simulink model "DroopandPImodel"  (R2024b)
settings: Solver=VariableStepAuto  StartTime=0.0  StopTime=10  RelTol=1e-3
values from neighbouring files (symbols this model uses):
  c = 160e-6    (= 0.00016)    [ParamTestSimulationDroop.m]    (also in ParamTestSimulatitestFirstandPI.m)
  deltaV = vrated*0.05    (= 5.5)    [ParamTestSimulationDroop.m]
  deltaW = 0.05*wrated    (= 18.8495559215)    [ParamTestSimulationDroop.m]
  Kp_currentLoop = X*r    (= 0.5)    [ParamTestSimulationDroop.m]    (also in ParamTestSimulatitestFirstandPI.m)
  Kp_voltageLoop = Xvoltage/Rc    (= 0.005)    [ParamTestSimulationDroop.m]    (also in ParamTestSimulatitestFirstandPI.m)
  l = 300e-6    (= 0.0003)    [ParamTestSimulationDroop.m]    (also in ParamTestSimulatitestFirstandPI.m)
  m = deltaW/Pnominal    (= 0.00628318530718)    [ParamTestSimulationDroop.m]
  n = deltaV/Qnominal    (= 0.011)    [ParamTestSimulationDroop.m]
  Pnominal = 3000    [ParamTestSimulationDroop.m]
  Qnominal = 500    [ParamTestSimulationDroop.m]
  r = 0.1    [ParamTestSimulationDroop.m]    (also in ParamTestSimulatitestFirstandPI.m)
  Rc = 1e3    (= 1000)    [ParamTestSimulationDroop.m]    (also in ParamTestSimulatitestFirstandPI.m)
  T32 = sqrt(2/3)*[1 0;-1/2 sqrt(3)/2;-1/2 -sqrt(3)/2]    [ParamTestSimulationDroop.m]    (also in ParamTestSimulatitestFirstandPI.m)
  towI_currentLoop = tow_currnet    (= 0.003)    [ParamTestSimulationDroop.m]    (also in ParamTestSimulatitestFirstandPI.m)
  towI_voltageLoop = tow_voltage    (= 0.16)    [ParamTestSimulationDroop.m]    (also in ParamTestSimulatitestFirstandPI.m)
  vrated = 110    [ParamTestSimulationDroop.m]
  wrated = 2*pi*60    (= 376.991118431)    [ParamTestSimulationDroop.m]
undefined symbols (not defined in the file or in its folder): DiscIntNeverNeededParam
libraries: spsThreePhaseSeriesRLCBranchLib x6, spsControlledVoltageSourceLib x3, spsThreePhaseVIMeasurementLib x2, spsGroundLib x1, sps_lib x1
settings Model: Creator=manip  LastModifiedBy=rashi
settings SolverCC: AlgebraicLoopSolver=TrustRegion
settings DebuggingCC: UnconnectedInputMsg=warning  UnconnectedOutputMsg=warning  UnconnectedLineMsg=warning
settings ModelReferenceCC: EnableRefExpFcnMdlSchedulingChecks=on
settings RTWCC: GPUComputeCapability=3.5

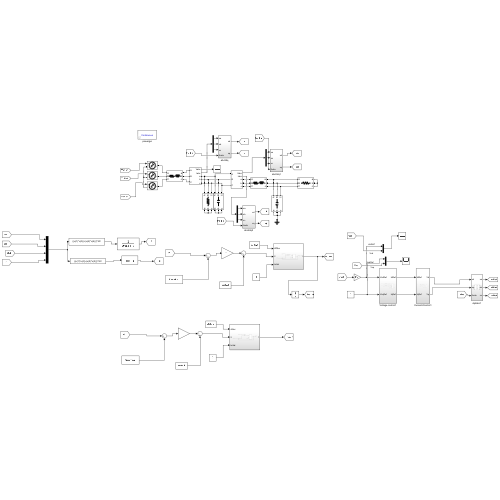
[thumbnail: Simulink's stored preview of the top-level diagram]
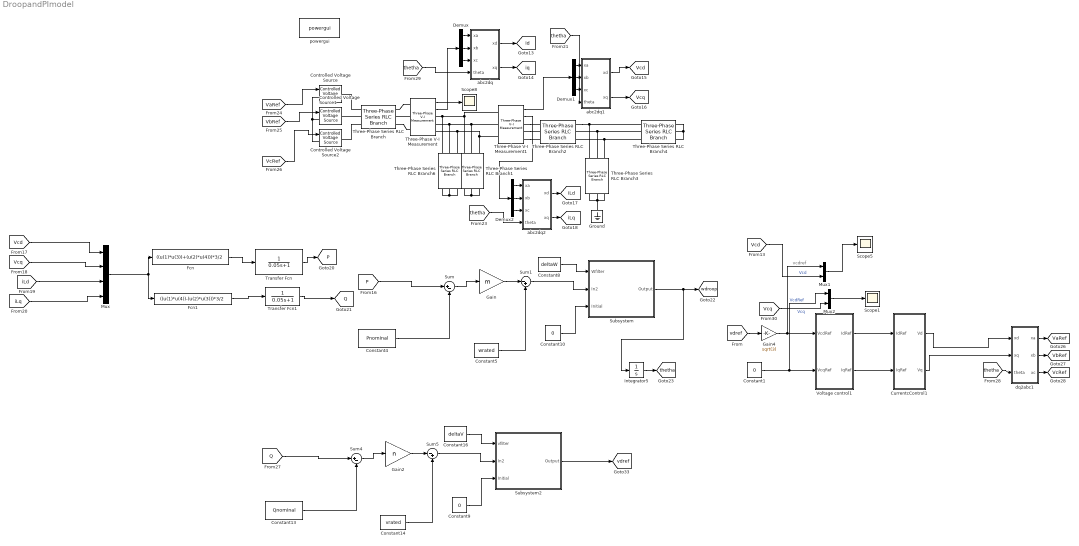
== system DroopandPImodel ==
  note: vcdref
  Constant1 : Constant  Value=0
  Constant10 : Constant  Value=0
  Constant13 : Constant  Value=Qnominal
  Constant14 : Constant  Value=vrated
  Constant16 : Constant  Value=deltaV
  Constant4 : Constant  Value=Pnominal
  Constant5 : Constant  Value=wrated
  Constant8 : Constant  Value=deltaW
  Constant9 : Constant  Value=0
  Controlled Voltage Source : spsControlledVoltageSourceLib/Controlled Voltage Source  Initialize=on  Source_Type=AC  Amplitude=0  Phase=0  Frequency=0  Measurements=None
  Controlled Voltage Source1 : spsControlledVoltageSourceLib/Controlled Voltage Source  Initialize=on  Source_Type=AC  Amplitude=0  Phase=0  Frequency=0  Measurements=None
  Controlled Voltage Source2 : spsControlledVoltageSourceLib/Controlled Voltage Source  Initialize=on  Source_Type=AC  Amplitude=0  Phase=0  Frequency=0  Measurements=None
  CurrentcControl1 : Subsystem
  Demux : Demux  Outputs=3
  Demux1 : Demux  Outputs=3
  Demux2 : Demux  Outputs=3
  Fcn : Fcn  Expr=((u(1)*u(3))+(u(2)*u(4)))*3/2
  Fcn1 : Fcn  Expr=((u(1)*u(4))-(u(2)*u(3)))*3/2
  Gain : Gain  Gain=m
  Gain2 : Gain  Gain=n
  Gain4 : Gain  Gain=sqrt(3)
  Ground : spsGroundLib/Ground  LConnTagsString=a
  Integrator5 : Integrator
  Mux : Mux
  Mux1 : Mux  Inputs=2
  Mux2 : Mux  Inputs=2
  Scope1 : Scope
  Scope5 : Scope
  Scope8 : Scope
  Subsystem : Subsystem
  Subsystem2 : Subsystem
  Sum : Sum  Inputs=|+-
  Sum1 : Sum  Inputs=|-+
  Sum4 : Sum  Inputs=|+-
  Sum5 : Sum  Inputs=|-+
  Three-Phase Series RLC Branch : spsThreePhaseSeriesRLCBranchLib/Three-Phase Series RLC Branch  LConnTagsString=A|B|C  RConnTagsString=A|B|C  BranchType=RL  Resistance=r  Inductance=l  Capacitance=1e-6  Measurements=None
  Three-Phase Series RLC Branch1 : spsThreePhaseSeriesRLCBranchLib/Three-Phase Series RLC Branch  LConnTagsString=A|B|C  RConnTagsString=A|B|C  BranchType=C  Resistance=r  Inductance=l  Capacitance=c  Measurements=None
  Three-Phase Series RLC Branch2 : spsThreePhaseSeriesRLCBranchLib/Three-Phase Series RLC Branch  LConnTagsString=A|B|C  RConnTagsString=A|B|C  BranchType=RL  Resistance=1  Inductance=4e-3  Capacitance=1e-6  Measurements=None
  Three-Phase Series RLC Branch3 : spsThreePhaseSeriesRLCBranchLib/Three-Phase Series RLC Branch  LConnTagsString=A|B|C  RConnTagsString=A|B|C  BranchType=C  Resistance=r  Inductance=l  Capacitance=1e-6  Measurements=None
  Three-Phase Series RLC Branch4 : spsThreePhaseSeriesRLCBranchLib/Three-Phase Series RLC Branch  LConnTagsString=A|B|C  RConnTagsString=A|B|C  BranchType=R  Resistance=50  Inductance=4e-3  Capacitance=1e-6  Measurements=None
  Three-Phase Series RLC Branch6 : spsThreePhaseSeriesRLCBranchLib/Three-Phase Series RLC Branch  LConnTagsString=A|B|C  RConnTagsString=A|B|C  BranchType=R  Resistance=Rc  Inductance=l  Capacitance=c  Measurements=None
  Three-Phase V-I Measurement : spsThreePhaseVIMeasurementLib/Three-Phase V-I Measurement  VoltageMeasurement=phase-to-ground  SetLabelV=off  LabelV=Vabc  Vpu=off  VpuLL=off  CurrentMeasurement=yes  SetLabelI=off  LabelI=Iabc  Ipu=off  Pbase=100e6  Vbase=500e3  OutputType=Complex  PhasorSimulation=off  PSBequivalent=0
  Three-Phase V-I Measurement1 : spsThreePhaseVIMeasurementLib/Three-Phase V-I Measurement  VoltageMeasurement=phase-to-ground  SetLabelV=off  LabelV=Vabc  Vpu=off  VpuLL=off  CurrentMeasurement=yes  SetLabelI=off  LabelI=Iabc  Ipu=off  Pbase=100e6  Vbase=500e3  OutputType=Complex  PhasorSimulation=off  PSBequivalent=0
  Transfer Fcn : TransferFcn  Denominator=[0.05 1]
  Transfer Fcn1 : TransferFcn  Denominator=[0.05 1]
  Voltage control1 : Subsystem
  abc2dq : Subsystem
  abc2dq1 : Subsystem
  abc2dq2 : Subsystem
  dq2abc1 : Subsystem
  powergui : sps_lib/powergui  Priority=1  SimulationMode=Continuous  SampleTime=50e-6  frequency=60  Iterations=50  frequencyindice=0  Pbase=100e6  ErrMax=1e-4  UnitsV=kV  UnitsW=MW  buscounter=0  FunctionMessages=off  echomessages=off  EnableUseOfTLC=off  CurrentSourceSwitches=off  DisableSnubberDevices=off  DisableRonSwitches=off  DisableVfSwitches=off  DisplayEquations=off  AutomaticDiscreteSolvers=off  SolverType=Tustin/Backward Euler (TBE)  Interpol=off  ExternalGateDelay=off  methode=off  Ts=100  x0status=blocks  SPID=on  SwTol=0  HookPort=off  NonlinearTolerance=1e-4  nMaxIteration=100  ContinueOnMaxIteration=off  RestoreLinks=warning  ResistiveCurrentMeasurement=off  Frange=[0:2:500]  Ylog=off  Xlog=on  ShowGrid=off  save=off  variable=ZData  structure=0  ZoomFFT=off  StartTime=0.0  cycles=1  DisplayStyle=1  fundamental=60  FreqAxis=off  MaxFrequency=1000  frequencyindicesteady=1  RmsSteady=1  display=off
  tag scope: P=global, Q=global, VaRef=global, VbRef=global, VcRef=global, Vcd=global, Vcq=global, iLd=global, iLq=global, id=global, iq=global, thetha=global, vdref=global, wdroop=global
  wires:
  Demux/1 -> abc2dq/1(xa)
  Demux/2 -> abc2dq/2(xb)
  Demux/3 -> abc2dq/3(xc)
  Three-Phase V-I Measurement/2 -> Demux/1
  abc2dq/1(xd) -> [id]
  abc2dq/2(xq) -> [iq]
  Three-Phase V-I Measurement1/1 -> Demux1/1
  Demux1/3 -> abc2dq1/3(xc)
  Demux1/2 -> abc2dq1/2(xb)
  Demux1/1 -> abc2dq1/1(xa)
  abc2dq1/1(xd) -> [Vcd]
  abc2dq1/2(xq) -> [Vcq]
  abc2dq2/2(xq) -> [iLq]
  abc2dq2/1(xd) -> [iLd]
  Three-Phase V-I Measurement1/2 -> Demux2/1
  Demux2/2 -> abc2dq2/2(xb)
  Demux2/3 -> abc2dq2/3(xc)
  Demux2/1 -> abc2dq2/1(xa)
  [iLd] -> Mux/3
  [iLq] -> Mux/4
  Mux/1 -> Fcn/1, Fcn1/1
  Constant4/1 -> Sum/2
  Sum/1 -> Gain/1
  Gain/1 -> Sum1/1
  Constant5/1 -> Sum1/2
  Sum1/1 -> Subsystem/2(In2)
  [VaRef] -> Controlled Voltage Source/1
  [VcRef] -> Controlled Voltage Source2/1
  dq2abc1/3(xc) -> [VcRef]
  CurrentcControl1/1(Vd) -> dq2abc1/1(xd)
  dq2abc1/2(xb) -> [VbRef]
  Constant1/1 -> Mux2/1, Voltage control1/2(VcqRef)
  dq2abc1/1(xa) -> [VaRef]
  CurrentcControl1/2(Vq) -> dq2abc1/2(xq)
  Subsystem/1(Output) -> Integrator5/1, [wdroop]
  Constant8/1 -> Subsystem/1(Wfilter)
  [VbRef] -> Controlled Voltage Source1/1
  [Vcd] -> Mux/1
  [Vcq] -> Mux/2
  Transfer Fcn/1 -> [P]
  Fcn/1 -> Transfer Fcn/1
  Fcn1/1 -> Transfer Fcn1/1
  Transfer Fcn1/1 -> [Q]
  [thetha] -> dq2abc1/3(theta)
  [thetha] -> abc2dq2/4(theta)
  Constant10/1 -> Subsystem/3(Initial)
  [P] -> Sum/1
  Constant9/1 -> Subsystem2/3(Initial)
  Constant16/1 -> Subsystem2/1(vfilter)
  Constant14/1 -> Sum5/2
  Constant13/1 -> Sum4/2
  Gain2/1 -> Sum5/1
  Sum5/1 -> Subsystem2/2(In2)
  Subsystem2/1(Output) -> [vdref]
  Sum4/1 -> Gain2/1
  [Q] -> Sum4/1
  Gain4/1 -> Voltage control1/1(VcdRef), Mux1/1  "VcdRef"
  [thetha] -> abc2dq/4(theta)
  [thetha] -> abc2dq1/4(theta)
  [vdref] -> Gain4/1
  Voltage control1/2(IqRef) -> CurrentcControl1/2(IqRef)
  Voltage control1/1(IdRef) -> CurrentcControl1/1(IdRef)
  [Vcd] -> Mux1/2  "Vcd"
  Mux2/1 -> Scope1/1
  [Vcq] -> Mux2/2  "Vcq"
  Mux1/1 -> Scope5/1
  Three-Phase V-I Measurement/1 -> Scope8/1
  Integrator5/1 -> [thetha]
  connections:
  Controlled Voltage Source1/LConn1 -- Controlled Voltage Source/LConn1 -- Controlled Voltage Source2/LConn1
  Three-Phase Series RLC Branch/LConn1 -- Controlled Voltage Source/RConn1
  Three-Phase Series RLC Branch/LConn2 -- Controlled Voltage Source1/RConn1
  Three-Phase Series RLC Branch/LConn3 -- Controlled Voltage Source2/RConn1
  Three-Phase V-I Measurement/LConn1 -- Three-Phase Series RLC Branch/RConn1
  Three-Phase V-I Measurement/LConn2 -- Three-Phase Series RLC Branch/RConn2
  Three-Phase Series RLC Branch/RConn3 -- Three-Phase V-I Measurement/LConn3
  Three-Phase Series RLC Branch1/RConn3 -- Three-Phase Series RLC Branch1/RConn2 -- Three-Phase Series RLC Branch1/RConn1
  Three-Phase Series RLC Branch1/LConn1 -- Three-Phase V-I Measurement1/LConn1 -- Three-Phase Series RLC Branch6/LConn1 -- Three-Phase V-I Measurement/RConn1
  Three-Phase V-I Measurement/RConn2 -- Three-Phase Series RLC Branch6/LConn2 -- Three-Phase V-I Measurement1/LConn2 -- Three-Phase Series RLC Branch1/LConn2
  Three-Phase V-I Measurement/RConn3 -- Three-Phase Series RLC Branch6/LConn3 -- Three-Phase V-I Measurement1/LConn3 -- Three-Phase Series RLC Branch1/LConn3
  Three-Phase V-I Measurement1/RConn1 -- Three-Phase Series RLC Branch2/LConn1
  Three-Phase V-I Measurement1/RConn2 -- Three-Phase Series RLC Branch2/LConn2
  Three-Phase V-I Measurement1/RConn3 -- Three-Phase Series RLC Branch2/LConn3
  Three-Phase Series RLC Branch3/RConn2 -- Three-Phase Series RLC Branch3/RConn3 -- Ground/LConn1 -- Three-Phase Series RLC Branch3/RConn1
  Three-Phase Series RLC Branch2/RConn1 -- Three-Phase Series RLC Branch3/LConn1 -- Three-Phase Series RLC Branch4/LConn1
  Three-Phase Series RLC Branch3/LConn2 -- Three-Phase Series RLC Branch2/RConn2 -- Three-Phase Series RLC Branch4/LConn2
  Three-Phase Series RLC Branch3/LConn3 -- Three-Phase Series RLC Branch4/LConn3 -- Three-Phase Series RLC Branch2/RConn3
  Three-Phase Series RLC Branch6/RConn3 -- Three-Phase Series RLC Branch6/RConn2 -- Three-Phase Series RLC Branch6/RConn1
  Three-Phase Series RLC Branch4/RConn1 -- Three-Phase Series RLC Branch4/RConn2 -- Three-Phase Series RLC Branch4/RConn3

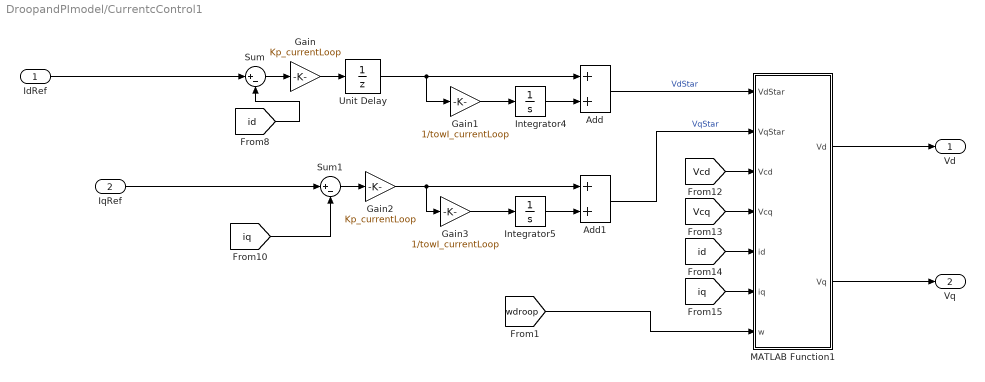
== system DroopandPImodel/CurrentcControl1 ==
  IdRef : Inport
  IqRef : Inport  Port=2
  Add : Sum
  Add1 : Sum
  Gain : Gain  Gain=Kp_currentLoop
  Gain1 : Gain  Gain=1/towI_currentLoop
  Gain2 : Gain  Gain=Kp_currentLoop
  Gain3 : Gain  Gain=1/towI_currentLoop
  Integrator4 : Integrator
  Integrator5 : Integrator
  MATLAB Function1 : MATLAB Function  TreatAsAtomicUnit=on
  Sum : Sum  Inputs=|+-
  Sum1 : Sum  Inputs=|+-
  Unit Delay : UnitDelay  SampleTime=1e-6  HasFrameUpgradeWarning=on
  Vd : Outport
  Vq : Outport  Port=2
  wires:
  [wdroop] -> MATLAB Function1/7(w)
  [iq] -> Sum1/2
  Add/1 -> MATLAB Function1/1(VdStar)  "VdStar"
  [Vcq] -> MATLAB Function1/4(Vcq)
  Gain2/1 -> Gain3/1, Add1/1
  IdRef/1 -> Sum/1
  [id] -> MATLAB Function1/5(id)
  Sum1/1 -> Gain2/1
  Gain3/1 -> Integrator5/1
  Sum/1 -> Gain/1
  IqRef/1 -> Sum1/1
  Add1/1 -> MATLAB Function1/2(VqStar)  "VqStar"
  Integrator5/1 -> Add1/2
  MATLAB Function1/2(Vq) -> Vq/1
  Gain/1 -> Unit Delay/1
  Integrator4/1 -> Add/2
  [Vcd] -> MATLAB Function1/3(Vcd)
  Gain1/1 -> Integrator4/1
  [id] -> Sum/2
  [iq] -> MATLAB Function1/6(iq)
  MATLAB Function1/1(Vd) -> Vd/1
  Unit Delay/1 -> Gain1/1, Add/1

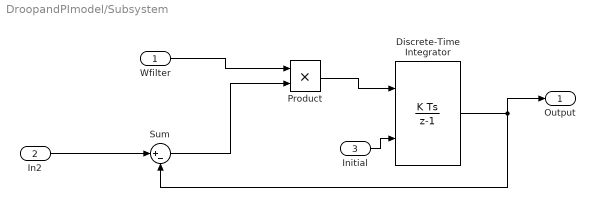
== system DroopandPImodel/Subsystem ==
  Wfilter : Inport
  In2 : Inport  Port=2
  Initial : Inport  Port=3
  Discrete-Time Integrator : DiscreteIntegrator  InitialConditionSource=external  SampleTime=1e-5  ICPrevOutput=DiscIntNeverNeededParam  ICPrevScaledInput=DiscIntNeverNeededParam
  Product : Product
  Sum : Sum  Inputs=|+-
  Output : Outport
  wires:
  Wfilter/1 -> Product/1
  In2/1 -> Sum/1
  Sum/1 -> Product/2
  Product/1 -> Discrete-Time Integrator/1
  Discrete-Time Integrator/1 -> Output/1, Sum/2
  Initial/1 -> Discrete-Time Integrator/2

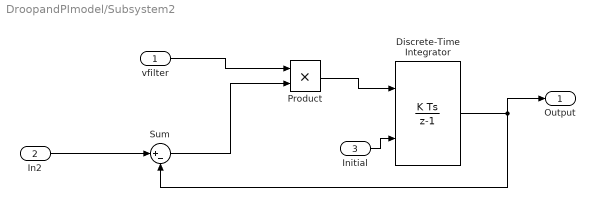
== system DroopandPImodel/Subsystem2 ==
  vfilter : Inport
  In2 : Inport  Port=2
  Initial : Inport  Port=3
  Discrete-Time Integrator : DiscreteIntegrator  InitialConditionSource=external  SampleTime=1e-5  ICPrevOutput=DiscIntNeverNeededParam  ICPrevScaledInput=DiscIntNeverNeededParam
  Product : Product
  Sum : Sum  Inputs=|+-
  Output : Outport
  wires:
  vfilter/1 -> Product/1
  In2/1 -> Sum/1
  Sum/1 -> Product/2
  Product/1 -> Discrete-Time Integrator/1
  Discrete-Time Integrator/1 -> Output/1, Sum/2
  Initial/1 -> Discrete-Time Integrator/2

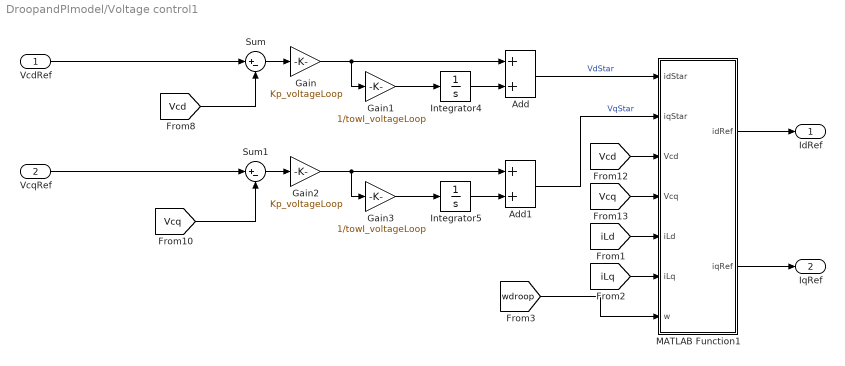
== system DroopandPImodel/Voltage control1 ==
  VcdRef : Inport
  VcqRef : Inport  Port=2
  Add : Sum
  Add1 : Sum
  Gain : Gain  Gain=Kp_voltageLoop
  Gain1 : Gain  Gain=1/towI_voltageLoop
  Gain2 : Gain  Gain=Kp_voltageLoop
  Gain3 : Gain  Gain=1/towI_voltageLoop
  Integrator4 : Integrator
  Integrator5 : Integrator
  MATLAB Function1 : MATLAB Function  TreatAsAtomicUnit=on
  Sum : Sum  Inputs=|+-
  Sum1 : Sum  Inputs=|+-
  IdRef : Outport
  IqRef : Outport  Port=2
  wires:
  Gain/1 -> Gain1/1, Add/1
  Integrator5/1 -> Add1/2
  VcqRef/1 -> Sum1/1
  Sum/1 -> Gain/1
  Gain3/1 -> Integrator5/1
  [iLd] -> MATLAB Function1/5(iLd)
  Sum1/1 -> Gain2/1
  VcdRef/1 -> Sum/1
  [Vcq] -> MATLAB Function1/4(Vcq)
  Gain2/1 -> Gain3/1, Add1/1
  [Vcd] -> Sum/2
  [iLq] -> MATLAB Function1/6(iLq)
  [wdroop] -> MATLAB Function1/7(w)
  Gain1/1 -> Integrator4/1
  [Vcq] -> Sum1/2
  Add1/1 -> MATLAB Function1/2(iqStar)  "VqStar"
  [Vcd] -> MATLAB Function1/3(Vcd)
  Add/1 -> MATLAB Function1/1(idStar)  "VdStar"
  Integrator4/1 -> Add/2
  MATLAB Function1/1(idRef) -> IdRef/1
  MATLAB Function1/2(iqRef) -> IqRef/1

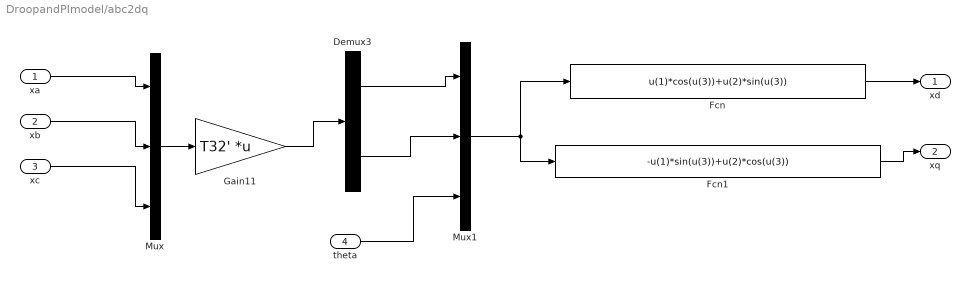
== system DroopandPImodel/abc2dq ==
  xa : Inport
  xb : Inport  Port=2
  xc : Inport  Port=3
  theta : Inport  Port=4
  Demux3 : Demux  Outputs=2
  Fcn : Fcn  Expr=u(1)*cos(u(3))+u(2)*sin(u(3))
  Fcn1 : Fcn  Expr=-u(1)*sin(u(3))+u(2)*cos(u(3))
  Gain11 : Gain  Gain=T32'  Multiplication=Matrix(K*u)
  Mux : Mux  Inputs=3
  Mux1 : Mux  Inputs=3
  xd : Outport
  xq : Outport  Port=2
  wires:
  Fcn1/1 -> xq/1
  theta/1 -> Mux1/3
  xb/1 -> Mux/2
  Mux/1 -> Gain11/1
  Gain11/1 -> Demux3/1
  xc/1 -> Mux/3
  Mux1/1 -> Fcn/1, Fcn1/1
  Fcn/1 -> xd/1
  xa/1 -> Mux/1
  Demux3/1 -> Mux1/1
  Demux3/2 -> Mux1/2

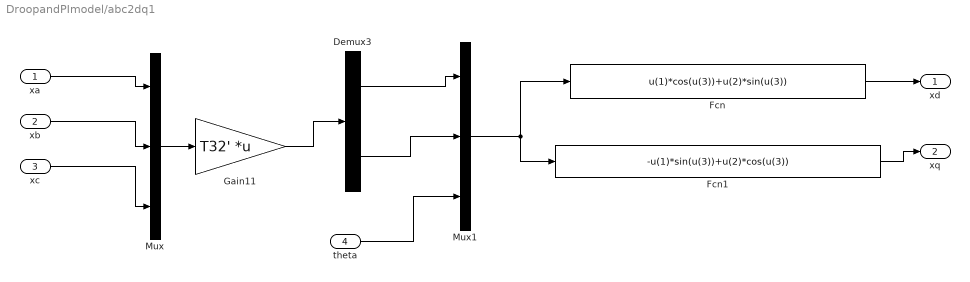
== system DroopandPImodel/abc2dq1 ==
  xa : Inport
  xb : Inport  Port=2
  xc : Inport  Port=3
  theta : Inport  Port=4
  Demux3 : Demux  Outputs=2
  Fcn : Fcn  Expr=u(1)*cos(u(3))+u(2)*sin(u(3))
  Fcn1 : Fcn  Expr=-u(1)*sin(u(3))+u(2)*cos(u(3))
  Gain11 : Gain  Gain=T32'  Multiplication=Matrix(K*u)
  Mux : Mux  Inputs=3
  Mux1 : Mux  Inputs=3
  xd : Outport
  xq : Outport  Port=2
  wires:
  Demux3/2 -> Mux1/2
  Demux3/1 -> Mux1/1
  xa/1 -> Mux/1
  Fcn/1 -> xd/1
  Mux1/1 -> Fcn1/1, Fcn/1
  xc/1 -> Mux/3
  Gain11/1 -> Demux3/1
  Mux/1 -> Gain11/1
  xb/1 -> Mux/2
  theta/1 -> Mux1/3
  Fcn1/1 -> xq/1

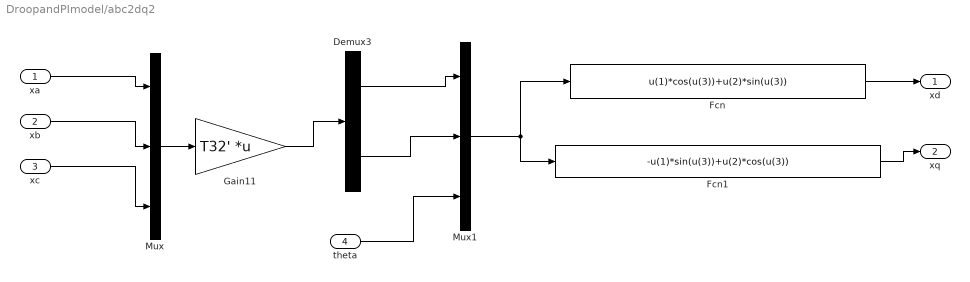
== system DroopandPImodel/abc2dq2 ==
  xa : Inport
  xb : Inport  Port=2
  xc : Inport  Port=3
  theta : Inport  Port=4
  Demux3 : Demux  Outputs=2
  Fcn : Fcn  Expr=u(1)*cos(u(3))+u(2)*sin(u(3))
  Fcn1 : Fcn  Expr=-u(1)*sin(u(3))+u(2)*cos(u(3))
  Gain11 : Gain  Gain=T32'  Multiplication=Matrix(K*u)
  Mux : Mux  Inputs=3
  Mux1 : Mux  Inputs=3
  xd : Outport
  xq : Outport  Port=2
  wires:
  Fcn1/1 -> xq/1
  theta/1 -> Mux1/3
  xb/1 -> Mux/2
  Mux/1 -> Gain11/1
  Gain11/1 -> Demux3/1
  xc/1 -> Mux/3
  Mux1/1 -> Fcn/1, Fcn1/1
  Fcn/1 -> xd/1
  xa/1 -> Mux/1
  Demux3/1 -> Mux1/1
  Demux3/2 -> Mux1/2

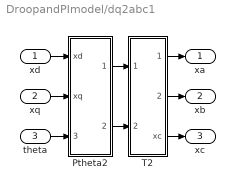
== system DroopandPImodel/dq2abc1 ==
  xd : Inport
  xq : Inport  Port=2
  theta : Inport  Port=3
  Ptheta2 : Subsystem
  T2 : Subsystem
  xa : Outport
  xb : Outport  Port=2
  xc : Outport  Port=3
  wires:
  xq/1 -> Ptheta2/2(xq)
  Ptheta2/2(xbeta) -> T2/2(xbeta)
  T2/1(xa) -> xa/1
  T2/3(xc) -> xc/1
  Ptheta2/1(xalpha) -> T2/1(xalpha)
  xd/1 -> Ptheta2/1(xd)
  theta/1 -> Ptheta2/3(theta)
  T2/2(xb) -> xb/1

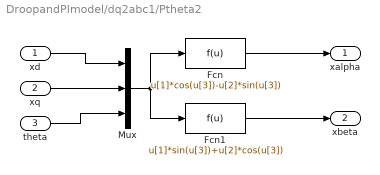
== system DroopandPImodel/dq2abc1/Ptheta2 ==
  xd : Inport
  xq : Inport  Port=2
  theta : Inport  Port=3
  Fcn : Fcn  Expr=u[1]*cos(u[3])-u[2]*sin(u[3])
  Fcn1 : Fcn  Expr=u[1]*sin(u[3])+u[2]*cos(u[3])
  Mux : Mux  Inputs=3
  xalpha : Outport
  xbeta : Outport  Port=2
  wires:
  xq/1 -> Mux/2
  xd/1 -> Mux/1
  Mux/1 -> Fcn1/1, Fcn/1
  Fcn1/1 -> xbeta/1
  Fcn/1 -> xalpha/1
  theta/1 -> Mux/3

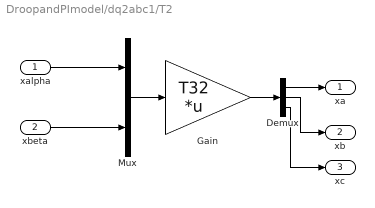
== system DroopandPImodel/dq2abc1/T2 ==
  xalpha : Inport
  xbeta : Inport  Port=2
  Demux : Demux  Outputs=3
  Gain : Gain  Gain=T32  Multiplication=Matrix(K*u)
  Mux : Mux  Inputs=2
  xa : Outport
  xb : Outport  Port=2
  xc : Outport  Port=3
  wires:
  Demux/3 -> xc/1
  Demux/2 -> xb/1
  Demux/1 -> xa/1
  Gain/1 -> Demux/1
  Mux/1 -> Gain/1
  xalpha/1 -> Mux/1
  xbeta/1 -> Mux/2

== matlab function DroopandPImodel/CurrentcControl1/MATLAB Function1 ==
  data: VdStar input; Vd output; VqStar input; Vcd input; Vcq input; id input; iq input; w input; Vq output; l parameter
function [Vd,Vq] = fcn(VdStar,VqStar,Vcd,Vcq,id,iq,w, l)

Vd = VdStar-l*w*iq+Vcd;
Vq = VqStar+l*w*id+Vcq;

== matlab function DroopandPImodel/Voltage control1/MATLAB Function1 ==
  data: idStar input; idRef output; iqStar input; Vcd input; Vcq input; iLd input; iLq input; w input; iqRef output; c parameter
function [idRef,iqRef] = fcn(idStar,iqStar,Vcd,Vcq,iLd,iLq,w, c)


idRef = idStar+iLd-c*w*Vcq;
iqRef = iqStar+iLq+c*w*Vcd;
